simulink library "lib_Transmission_Simscape_1"  (R2017a)
settings: Solver=VariableStepAuto  StartTime=0.0  StopTime=10.0  RelTol=1e-3
libraries: fl_lib x32, sdl_lib x12, nesl_utility x4
settings Model: Creator=Di Russo  LastModifiedBy=Di Russo

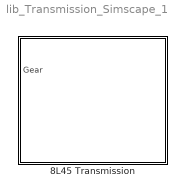
== system lib_Transmission_Simscape_1 ==
  8L45 Transmission : Subsystem  AncestorBlock=EcoCAR3_Lib/6L45 Transmission

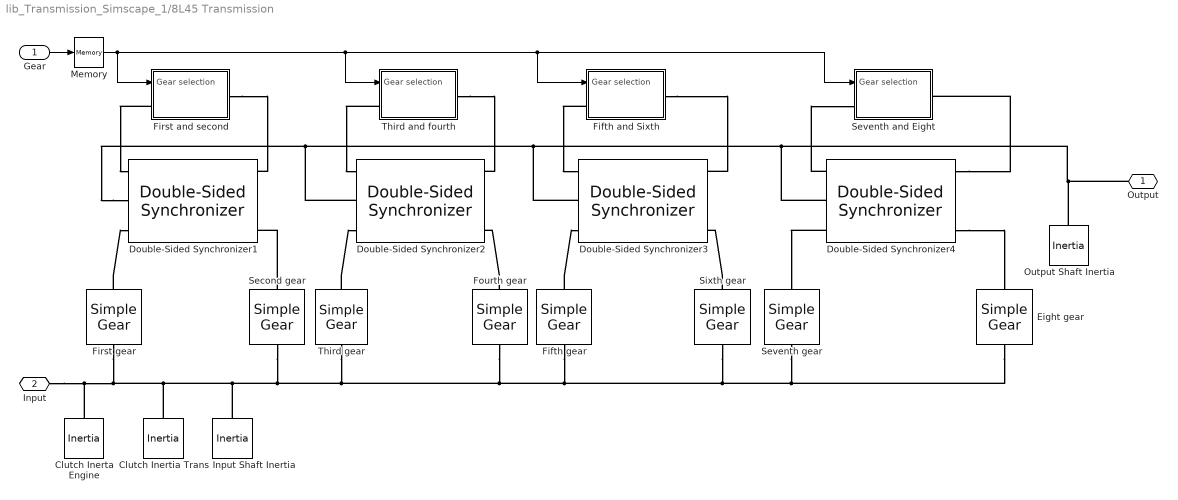
== system lib_Transmission_Simscape_1/8L45 Transmission ==
  Gear : Inport
  Clutch Inerta Engine : fl_lib/Mechanical/Rotational Elements/Inertia  inertia=Gearbox.ClutchInertiaEngine kg*m^2  w_specify=off  w_priority=High  w=580*2*pi/60 rad/s  w_nominal_specify=off  w_nominal_unit=rad/s  w_nominal_value=1  t_specify=off  t_priority=High  t=0 N*m  t_nominal_specify=off  t_nominal_unit=N*m  t_nominal_value=1
  Clutch Inertia Trans : fl_lib/Mechanical/Rotational Elements/Inertia  inertia=Gearbox.ClutchInertiaTrans kg*m^2  w_specify=off  w_priority=High  w=580*2*pi/60 rad/s  w_nominal_specify=off  w_nominal_unit=rad/s  w_nominal_value=1  t_specify=off  t_priority=High  t=0 N*m  t_nominal_specify=off  t_nominal_unit=N*m  t_nominal_value=1
  Double-Sided Synchronizer{1..4} (4 alike) : sdl_lib/Clutches/Double-Sided Synchronizer  model=1  max_torque=1000 N*m  n_teeth=6  clutch_backlash=10 deg  radius=200 mm  clutch_stiffness=1e+7 N*m/rad  clutch_damping=100 N*m/(rad/s)  fric_coeff=0.05  engagement_speed=Inf rad/s  d_o=150 mm  d_i=100 mm  theta=12 deg  friction_model=1  mu_coulomb=0.3  mu_w_vector=[ 0 0.1 0.2 0.3 0.4 0.5 1 2 5 10 100 1000 ] rad/s  mu_coulomb_vector=[ 0.29 0.28 0.26 0.22 0.21 0.2 0.2 0.19 0.19 0.19 0.19 0.19 ]  mu_interp_method=1  mu_extrap_method=1  mu_static=0.35  w_tol=0.001 rad/s  force_min=1 N  peak_force=100 N  width=3 mm  detent_visc_fric_transl=0.1 N/(m/s)  friction_ratio=0.01  v_thr=0.05 m/s  dog_clutch_ring_hub_gap=5 mm  engagement_overlap=3 mm  tooth_height=10 mm  cone_clutch_ring_hub_gap=3 mm  dog_clutch_transl_stiffness=1e+6 N/m  cone_clutch_transl_stiffness=1e+6 N/m  dog_clutch_transl_damping=1000 N/(m/s)  cone_clutch_transl_damping=1000 N/(m/s)  dog_clutch_visc_fric_transl=100 N/(m/s)  initial_state_locked=3  dog_clutch_init_pos=0 mm  cone_clutch_init_pos=0 mm  init_rel_angle_A=0 deg  init_rel_angle_B=0 deg  torque_temperature_TLU=[280.0, 300.0, 320.0] K  max_torque_vector=[1000.0, 1050.0, 1000.0] N*m  torque_interp_method=1  torque_extrap_method=1  mu_temperature_TLU=[280.0, 300.0, 320.0] K  mu_coulomb_temp_vector=[0.3, 0.28, 0.25]  mu_coulomb_matrix=[0.34, 0.32, 0.3; 0.3, 0.28, 0.25; 0.25, 0.2, 0.15]  mu_static_vector=[0.4, 0.38, 0.36]  thermal_mass=100 kJ/K  T_init=300 K
      settings: SourceProductName=Simscape Driveline  SourceProductBaseCode=LD
  Eight gear : sdl_lib/Gears/Simple Gear  ratio=GearBox.L45.gr6  rotation_direction=1  friction_model=1  T_noload=0.1 N*m  T_nom=5 N*m  efficiency_nom=0.8  efficiency=0.8  mu_visc=[ 0.01 0.01 ] N*m/(rad/s)  w_thr=0.01 rad/s  pwr_thr=0.001 W  temperature_TLU=[280.0, 300.0, 320.0] K  load_TLU=[1.0, 5.0, 10.0] N*m  efficiency_TLU=[0.95, 0.9, 0.85]  efficiency_TLU2=[0.85, 0.8, 0.75; 0.95, 0.9, 0.85; 0.85, 0.8, 0.7]  thermal_mass=50 J/K  T_init=300 K
      settings: SourceProductName=Simscape Driveline
  Fifth gear : sdl_lib/Gears/Simple Gear  ratio=GearBox.L45.gr5  rotation_direction=1  friction_model=1  T_noload=0.1 N*m  T_nom=5 N*m  efficiency_nom=0.8  efficiency=0.8  mu_visc=[ 0.01 0.01 ] N*m/(rad/s)  w_thr=0.01 rad/s  pwr_thr=0.001 W  temperature_TLU=[280.0, 300.0, 320.0] K  load_TLU=[1.0, 5.0, 10.0] N*m  efficiency_TLU=[0.95, 0.9, 0.85]  efficiency_TLU2=[0.85, 0.8, 0.75; 0.95, 0.9, 0.85; 0.85, 0.8, 0.7]  thermal_mass=50 J/K  T_init=300 K
      settings: SourceProductName=Simscape Driveline
  Fifth and Sixth : Subsystem
  First gear : sdl_lib/Gears/Simple Gear  ratio=GearBox.L45.gr1  rotation_direction=1  friction_model=1  T_noload=0.1 N*m  T_nom=5 N*m  efficiency_nom=0.8  efficiency=0.8  mu_visc=[ 0.01 0.01 ] N*m/(rad/s)  w_thr=0.01 rad/s  pwr_thr=0.001 W  temperature_TLU=[280.0, 300.0, 320.0] K  load_TLU=[1.0, 5.0, 10.0] N*m  efficiency_TLU=[0.95, 0.9, 0.85]  efficiency_TLU2=[0.85, 0.8, 0.75; 0.95, 0.9, 0.85; 0.85, 0.8, 0.7]  thermal_mass=50 J/K  T_init=300 K
      settings: SourceProductName=Simscape Driveline
  First and second : Subsystem
  Fourth gear : sdl_lib/Gears/Simple Gear  ratio=GearBox.L45.gr4  rotation_direction=1  friction_model=1  T_noload=0.1 N*m  T_nom=5 N*m  efficiency_nom=0.8  efficiency=0.8  mu_visc=[ 0.01 0.01 ] N*m/(rad/s)  w_thr=0.01 rad/s  pwr_thr=0.001 W  temperature_TLU=[280.0, 300.0, 320.0] K  load_TLU=[1.0, 5.0, 10.0] N*m  efficiency_TLU=[0.95, 0.9, 0.85]  efficiency_TLU2=[0.85, 0.8, 0.75; 0.95, 0.9, 0.85; 0.85, 0.8, 0.7]  thermal_mass=50 J/K  T_init=300 K
      settings: SourceProductName=Simscape Driveline
  Input Shaft Inertia : fl_lib/Mechanical/Rotational Elements/Inertia  inertia=Gearbox.InputShaftInertia kg*m^2  w_specify=off  w_priority=High  w=580*2*pi/60 rad/s  w_nominal_specify=off  w_nominal_unit=rad/s  w_nominal_value=1  t_specify=off  t_priority=High  t=0 N*m  t_nominal_specify=off  t_nominal_unit=N*m  t_nominal_value=1
  Memory : Memory
  Output Shaft Inertia : fl_lib/Mechanical/Rotational Elements/Inertia  inertia=Gearbox.OutputShaftInertia kg*m^2  w_specify=off  w_priority=High  w=580*2*pi/60 rad/s  w_nominal_specify=off  w_nominal_unit=rad/s  w_nominal_value=1  t_specify=off  t_priority=High  t=0 N*m  t_nominal_specify=off  t_nominal_unit=N*m  t_nominal_value=1
  Second gear : sdl_lib/Gears/Simple Gear  ratio=GearBox.L45.gr2  rotation_direction=1  friction_model=1  T_noload=0.1 N*m  T_nom=5 N*m  efficiency_nom=0.8  efficiency=0.8  mu_visc=[ 0.01 0.01 ] N*m/(rad/s)  w_thr=0.01 rad/s  pwr_thr=0.001 W  temperature_TLU=[280.0, 300.0, 320.0] K  load_TLU=[1.0, 5.0, 10.0] N*m  efficiency_TLU=[0.95, 0.9, 0.85]  efficiency_TLU2=[0.85, 0.8, 0.75; 0.95, 0.9, 0.85; 0.85, 0.8, 0.7]  thermal_mass=50 J/K  T_init=300 K
      settings: SourceProductName=Simscape Driveline
  Seventh gear : sdl_lib/Gears/Simple Gear  ratio=GearBox.L45.gr6  rotation_direction=1  friction_model=1  T_noload=0.1 N*m  T_nom=5 N*m  efficiency_nom=0.8  efficiency=0.8  mu_visc=[ 0.01 0.01 ] N*m/(rad/s)  w_thr=0.01 rad/s  pwr_thr=0.001 W  temperature_TLU=[280.0, 300.0, 320.0] K  load_TLU=[1.0, 5.0, 10.0] N*m  efficiency_TLU=[0.95, 0.9, 0.85]  efficiency_TLU2=[0.85, 0.8, 0.75; 0.95, 0.9, 0.85; 0.85, 0.8, 0.7]  thermal_mass=50 J/K  T_init=300 K
      settings: SourceProductName=Simscape Driveline
  Seventh and Eight : Subsystem
  Sixth gear : sdl_lib/Gears/Simple Gear  ratio=GearBox.L45.gr6  rotation_direction=1  friction_model=1  T_noload=0.1 N*m  T_nom=5 N*m  efficiency_nom=0.8  efficiency=0.8  mu_visc=[ 0.01 0.01 ] N*m/(rad/s)  w_thr=0.01 rad/s  pwr_thr=0.001 W  temperature_TLU=[280.0, 300.0, 320.0] K  load_TLU=[1.0, 5.0, 10.0] N*m  efficiency_TLU=[0.95, 0.9, 0.85]  efficiency_TLU2=[0.85, 0.8, 0.75; 0.95, 0.9, 0.85; 0.85, 0.8, 0.7]  thermal_mass=50 J/K  T_init=300 K
      settings: SourceProductName=Simscape Driveline
  Third gear : sdl_lib/Gears/Simple Gear  ratio=GearBox.L45.gr3  rotation_direction=1  friction_model=1  T_noload=0.1 N*m  T_nom=5 N*m  efficiency_nom=0.8  efficiency=0.8  mu_visc=[ 0.01 0.01 ] N*m/(rad/s)  w_thr=0.01 rad/s  pwr_thr=0.001 W  temperature_TLU=[280.0, 300.0, 320.0] K  load_TLU=[1.0, 5.0, 10.0] N*m  efficiency_TLU=[0.95, 0.9, 0.85]  efficiency_TLU2=[0.85, 0.8, 0.75; 0.95, 0.9, 0.85; 0.85, 0.8, 0.7]  thermal_mass=50 J/K  T_init=300 K
      settings: SourceProductName=Simscape Driveline
  Third and fourth : Subsystem
  Output : PMIOPort  Port=1  Side=Right
  Input : PMIOPort  Port=2  Side=Left
  wires:
  Memory/1 -> Third and fourth/1(Gear selection), Seventh and Eight/1(Gear selection), Fifth and Sixth/1(Gear selection), First and second/1(Gear selection)
  Gear/1 -> Memory/1
  connections:
  Sixth gear/RConn1 -- Double-Sided Synchronizer3/RConn3
  Third and fourth/RConn1 -- Double-Sided Synchronizer2/RConn1
  First and second/RConn1 -- Double-Sided Synchronizer1/RConn1
  Double-Sided Synchronizer1/LConn2 -- Double-Sided Synchronizer2/LConn2 -- Double-Sided Synchronizer3/LConn2 -- Output/RConn1 -- Output Shaft Inertia/LConn1 -- Double-Sided Synchronizer4/LConn2
  Clutch Inertia Trans/LConn1 -- First gear/LConn1 -- Clutch Inerta Engine/LConn1 -- Input/RConn1 -- Input Shaft Inertia/LConn1 -- Second gear/LConn1 -- Third gear/LConn1 -- Fourth gear/LConn1 -- Fifth gear/LConn1 -- Sixth gear/LConn1 -- Eight gear/LConn1 -- Seventh gear/LConn1
  Fifth and Sixth/RConn1 -- Double-Sided Synchronizer3/RConn1
  Fifth and Sixth/LConn1 -- Double-Sided Synchronizer3/LConn1
  Third and fourth/LConn1 -- Double-Sided Synchronizer2/LConn1
  Fourth gear/RConn1 -- Double-Sided Synchronizer2/RConn3
  Fifth gear/RConn1 -- Double-Sided Synchronizer3/LConn3
  Second gear/RConn1 -- Double-Sided Synchronizer1/RConn3
  Third gear/RConn1 -- Double-Sided Synchronizer2/LConn3
  First gear/RConn1 -- Double-Sided Synchronizer1/LConn3
  First and second/LConn1 -- Double-Sided Synchronizer1/LConn1
  Double-Sided Synchronizer4/LConn3 -- Seventh gear/RConn1
  Double-Sided Synchronizer4/RConn3 -- Eight gear/RConn1
  Double-Sided Synchronizer4/LConn1 -- Seventh and Eight/LConn1
  Double-Sided Synchronizer4/RConn1 -- Seventh and Eight/RConn1

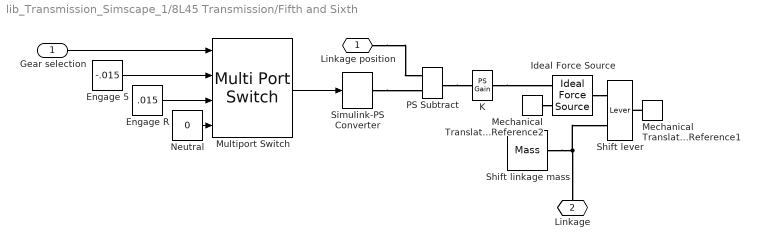
== system lib_Transmission_Simscape_1/8L45 Transmission/Fifth and Sixth ==
  Gear selection : Inport
  Engage 5 : Constant  Value=-.015
  Engage R : Constant  Value=.015
  Ideal Force Source : fl_lib/Mechanical/Mechanical Sources/Ideal Force Source
  K : fl_lib/Physical Signals/Functions/PS Gain  gain=750
  Mechanical Translational Reference1 : fl_lib/Mechanical/Translational Elements/Mechanical Translational Reference
  Mechanical Translational Reference2 : fl_lib/Mechanical/Translational Elements/Mechanical Translational Reference
  Multiport Switch : MultiPortSwitch  DataPortOrder=Specify indices  DataPortIndices={5,6}  DataPortForDefault=Additional data port  DiagnosticForDefault=None
  Neutral : Constant  Value=0
  PS Subtract : fl_lib/Physical Signals/Functions/PS Subtract
      settings: SourceProductName=Simscape
  Shift lever : fl_lib/Mechanical/Mechanisms/Lever  arm_AC=0.1 m  arm_BC=0.02 m  f_A_specify=off  f_A_priority=High  f_A=0 N  f_A_nominal_specify=off  f_A_nominal_unit=N  f_A_nominal_value=1  f_B_specify=off  f_B_priority=High  f_B=0 N  f_B_nominal_specify=off  f_B_nominal_unit=N  f_B_nominal_value=1  f_C_specify=off  f_C_priority=High  f_C=0 N  f_C_nominal_specify=off  f_C_nominal_unit=N  f_C_nominal_value=1
      settings: SourceProductName=Simscape  SourceProductBaseCode=SS
  Shift linkage mass : fl_lib/Mechanical/Translational Elements/Mass  mass=1 kg  v_specify=on  v_priority=High  v=0 m/s  v_nominal_specify=off  v_nominal_unit=m/s  v_nominal_value=1  f_specify=off  f_priority=High  f=0 N  f_nominal_specify=off  f_nominal_unit=N  f_nominal_value=1
  Simulink-PS Converter : nesl_utility/Simulink-PS Converter  PhysicalDomain=network_engine_domain  SubClassName=ps_input  LeftPortType=input  RightPortType=output  PseudoPeriodic=off  Frequencies=[]  NoiseDistribution=none  NoiseParameters=[]  Unit=1  AffineConversion=off  FilteringAndDerivatives=filter  SimscapeFilterOrder=1  InputFilterTimeConstant=.001  UdotUserProvided=1
  Linkage position : PMIOPort  Port=1  Side=Right
  Linkage : PMIOPort  Port=2  Side=Left
  wires:
  Gear selection/1 -> Multiport Switch/1
  Engage 5/1 -> Multiport Switch/2
  Engage R/1 -> Multiport Switch/3
  Neutral/1 -> Multiport Switch/4
  Multiport Switch/1 -> Simulink-PS Converter/1
  connections:
  K/RConn1 -- Ideal Force Source/RConn1
  Linkage position/RConn1 -- PS Subtract/LConn1
  Simulink-PS Converter/RConn1 -- PS Subtract/LConn2
  Ideal Force Source/LConn1 -- Shift lever/LConn1
  Mechanical Translational Reference1/LConn1 -- Shift lever/RConn1
  Mechanical Translational Reference2/LConn1 -- Ideal Force Source/RConn2
  Shift linkage mass/LConn1 -- Shift lever/LConn2 -- Linkage/RConn1
  PS Subtract/RConn1 -- K/LConn1

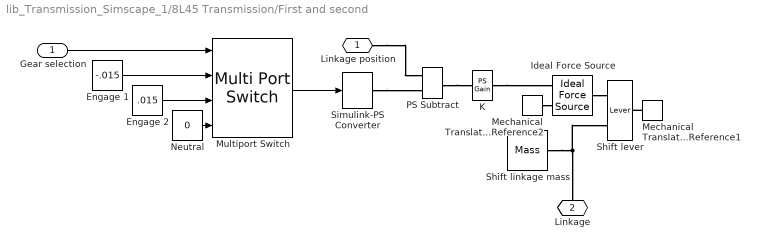
== system lib_Transmission_Simscape_1/8L45 Transmission/First and second ==
  Gear selection : Inport
  Engage 1 : Constant  Value=-.015
  Engage 2 : Constant  Value=.015
  Ideal Force Source : fl_lib/Mechanical/Mechanical Sources/Ideal Force Source
  K : fl_lib/Physical Signals/Functions/PS Gain  gain=750
  Mechanical Translational Reference1 : fl_lib/Mechanical/Translational Elements/Mechanical Translational Reference
  Mechanical Translational Reference2 : fl_lib/Mechanical/Translational Elements/Mechanical Translational Reference
  Multiport Switch : MultiPortSwitch  DataPortOrder=Specify indices  DataPortIndices={1,2}  DataPortForDefault=Additional data port  DiagnosticForDefault=None
  Neutral : Constant  Value=0
  PS Subtract : fl_lib/Physical Signals/Functions/PS Subtract
      settings: SourceProductName=Simscape
  Shift lever : fl_lib/Mechanical/Mechanisms/Lever  arm_AC=0.1 m  arm_BC=0.02 m  f_A_specify=off  f_A_priority=High  f_A=0 N  f_A_nominal_specify=off  f_A_nominal_unit=N  f_A_nominal_value=1  f_B_specify=off  f_B_priority=High  f_B=0 N  f_B_nominal_specify=off  f_B_nominal_unit=N  f_B_nominal_value=1  f_C_specify=off  f_C_priority=High  f_C=0 N  f_C_nominal_specify=off  f_C_nominal_unit=N  f_C_nominal_value=1
      settings: SourceProductName=Simscape  SourceProductBaseCode=SS
  Shift linkage mass : fl_lib/Mechanical/Translational Elements/Mass  mass=1 kg  v_specify=on  v_priority=High  v=0 m/s  v_nominal_specify=off  v_nominal_unit=m/s  v_nominal_value=1  f_specify=off  f_priority=High  f=0 N  f_nominal_specify=off  f_nominal_unit=N  f_nominal_value=1
  Simulink-PS Converter : nesl_utility/Simulink-PS Converter  PhysicalDomain=network_engine_domain  SubClassName=ps_input  LeftPortType=input  RightPortType=output  PseudoPeriodic=off  Frequencies=[]  NoiseDistribution=none  NoiseParameters=[]  Unit=1  AffineConversion=off  FilteringAndDerivatives=filter  SimscapeFilterOrder=1  InputFilterTimeConstant=.001  UdotUserProvided=1
  Linkage position : PMIOPort  Port=1  Side=Right
  Linkage : PMIOPort  Port=2  Side=Left
  wires:
  Gear selection/1 -> Multiport Switch/1
  Engage 1/1 -> Multiport Switch/2
  Engage 2/1 -> Multiport Switch/3
  Neutral/1 -> Multiport Switch/4
  Multiport Switch/1 -> Simulink-PS Converter/1
  connections:
  K/RConn1 -- Ideal Force Source/RConn1
  Linkage position/RConn1 -- PS Subtract/LConn1
  Simulink-PS Converter/RConn1 -- PS Subtract/LConn2
  Ideal Force Source/LConn1 -- Shift lever/LConn1
  Mechanical Translational Reference1/LConn1 -- Shift lever/RConn1
  Mechanical Translational Reference2/LConn1 -- Ideal Force Source/RConn2
  Shift linkage mass/LConn1 -- Shift lever/LConn2 -- Linkage/RConn1
  PS Subtract/RConn1 -- K/LConn1

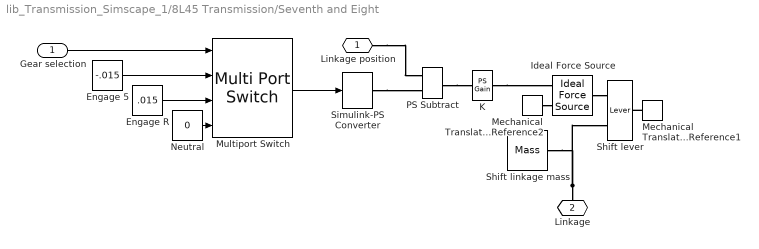
== system lib_Transmission_Simscape_1/8L45 Transmission/Seventh and Eight ==
  Gear selection : Inport
  Engage 5 : Constant  Value=-.015
  Engage R : Constant  Value=.015
  Ideal Force Source : fl_lib/Mechanical/Mechanical Sources/Ideal Force Source
  K : fl_lib/Physical Signals/Functions/PS Gain  gain=750
  Mechanical Translational Reference1 : fl_lib/Mechanical/Translational Elements/Mechanical Translational Reference
  Mechanical Translational Reference2 : fl_lib/Mechanical/Translational Elements/Mechanical Translational Reference
  Multiport Switch : MultiPortSwitch  DataPortOrder=Specify indices  DataPortIndices={5,6}  DataPortForDefault=Additional data port  DiagnosticForDefault=None
  Neutral : Constant  Value=0
  PS Subtract : fl_lib/Physical Signals/Functions/PS Subtract
      settings: SourceProductName=Simscape
  Shift lever : fl_lib/Mechanical/Mechanisms/Lever  arm_AC=0.1 m  arm_BC=0.02 m  f_A_specify=off  f_A_priority=High  f_A=0 N  f_A_nominal_specify=off  f_A_nominal_unit=N  f_A_nominal_value=1  f_B_specify=off  f_B_priority=High  f_B=0 N  f_B_nominal_specify=off  f_B_nominal_unit=N  f_B_nominal_value=1  f_C_specify=off  f_C_priority=High  f_C=0 N  f_C_nominal_specify=off  f_C_nominal_unit=N  f_C_nominal_value=1
      settings: SourceProductName=Simscape  SourceProductBaseCode=SS
  Shift linkage mass : fl_lib/Mechanical/Translational Elements/Mass  mass=1 kg  v_specify=on  v_priority=High  v=0 m/s  v_nominal_specify=off  v_nominal_unit=m/s  v_nominal_value=1  f_specify=off  f_priority=High  f=0 N  f_nominal_specify=off  f_nominal_unit=N  f_nominal_value=1
  Simulink-PS Converter : nesl_utility/Simulink-PS Converter  PhysicalDomain=network_engine_domain  SubClassName=ps_input  LeftPortType=input  RightPortType=output  PseudoPeriodic=off  Frequencies=[]  NoiseDistribution=none  NoiseParameters=[]  Unit=1  AffineConversion=off  FilteringAndDerivatives=filter  SimscapeFilterOrder=1  InputFilterTimeConstant=.001  UdotUserProvided=1
  Linkage position : PMIOPort  Port=1  Side=Right
  Linkage : PMIOPort  Port=2  Side=Left
  wires:
  Multiport Switch/1 -> Simulink-PS Converter/1
  Neutral/1 -> Multiport Switch/4
  Engage R/1 -> Multiport Switch/3
  Engage 5/1 -> Multiport Switch/2
  Gear selection/1 -> Multiport Switch/1
  connections:
  PS Subtract/RConn1 -- K/LConn1
  Linkage/RConn1 -- Shift lever/LConn2 -- Shift linkage mass/LConn1
  Mechanical Translational Reference2/LConn1 -- Ideal Force Source/RConn2
  Mechanical Translational Reference1/LConn1 -- Shift lever/RConn1
  Ideal Force Source/LConn1 -- Shift lever/LConn1
  Simulink-PS Converter/RConn1 -- PS Subtract/LConn2
  Linkage position/RConn1 -- PS Subtract/LConn1
  K/RConn1 -- Ideal Force Source/RConn1

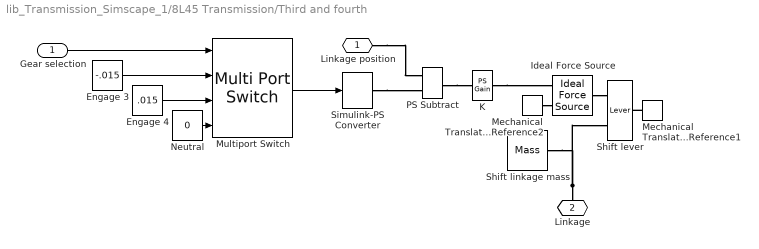
== system lib_Transmission_Simscape_1/8L45 Transmission/Third and fourth ==
  Gear selection : Inport
  Engage 3 : Constant  Value=-.015
  Engage 4 : Constant  Value=.015
  Ideal Force Source : fl_lib/Mechanical/Mechanical Sources/Ideal Force Source
  K : fl_lib/Physical Signals/Functions/PS Gain  gain=750
  Mechanical Translational Reference1 : fl_lib/Mechanical/Translational Elements/Mechanical Translational Reference
  Mechanical Translational Reference2 : fl_lib/Mechanical/Translational Elements/Mechanical Translational Reference
  Multiport Switch : MultiPortSwitch  DataPortOrder=Specify indices  DataPortIndices={3,4}  DataPortForDefault=Additional data port  DiagnosticForDefault=None
  Neutral : Constant  Value=0
  PS Subtract : fl_lib/Physical Signals/Functions/PS Subtract
      settings: SourceProductName=Simscape
  Shift lever : fl_lib/Mechanical/Mechanisms/Lever  arm_AC=0.1 m  arm_BC=0.02 m  f_A_specify=off  f_A_priority=High  f_A=0 N  f_A_nominal_specify=off  f_A_nominal_unit=N  f_A_nominal_value=1  f_B_specify=off  f_B_priority=High  f_B=0 N  f_B_nominal_specify=off  f_B_nominal_unit=N  f_B_nominal_value=1  f_C_specify=off  f_C_priority=High  f_C=0 N  f_C_nominal_specify=off  f_C_nominal_unit=N  f_C_nominal_value=1
      settings: SourceProductName=Simscape  SourceProductBaseCode=SS
  Shift linkage mass : fl_lib/Mechanical/Translational Elements/Mass  mass=1 kg  v_specify=on  v_priority=High  v=0 m/s  v_nominal_specify=off  v_nominal_unit=m/s  v_nominal_value=1  f_specify=off  f_priority=High  f=0 N  f_nominal_specify=off  f_nominal_unit=N  f_nominal_value=1
  Simulink-PS Converter : nesl_utility/Simulink-PS Converter  PhysicalDomain=network_engine_domain  SubClassName=ps_input  LeftPortType=input  RightPortType=output  PseudoPeriodic=off  Frequencies=[]  NoiseDistribution=none  NoiseParameters=[]  Unit=1  AffineConversion=off  FilteringAndDerivatives=filter  SimscapeFilterOrder=1  InputFilterTimeConstant=.001  UdotUserProvided=1
  Linkage position : PMIOPort  Port=1  Side=Right
  Linkage : PMIOPort  Port=2  Side=Left
  wires:
  Multiport Switch/1 -> Simulink-PS Converter/1
  Neutral/1 -> Multiport Switch/4
  Engage 4/1 -> Multiport Switch/3
  Engage 3/1 -> Multiport Switch/2
  Gear selection/1 -> Multiport Switch/1
  connections:
  PS Subtract/RConn1 -- K/LConn1
  Linkage/RConn1 -- Shift lever/LConn2 -- Shift linkage mass/LConn1
  Mechanical Translational Reference2/LConn1 -- Ideal Force Source/RConn2
  Mechanical Translational Reference1/LConn1 -- Shift lever/RConn1
  Ideal Force Source/LConn1 -- Shift lever/LConn1
  Simulink-PS Converter/RConn1 -- PS Subtract/LConn2
  Linkage position/RConn1 -- PS Subtract/LConn1
  K/RConn1 -- Ideal Force Source/RConn1
